simulink model "Echantillon"  (R2023b)
settings: Solver=VariableStepAuto  StartTime=0.0  StopTime=10.0  RelTol=1e-3
values from neighbouring files (symbols this model uses):
  C2 = retard/sysbod2(1 - retard)    [script_TD_asser_echantZdan.m]
  sysbod1 = c2d(sysbo , Te , 'foh')    [script_TD_asser_echantZdan.m]
libraries: slctrl_linear x1
settings Model: Creator=boris  LastModifiedBy=boris

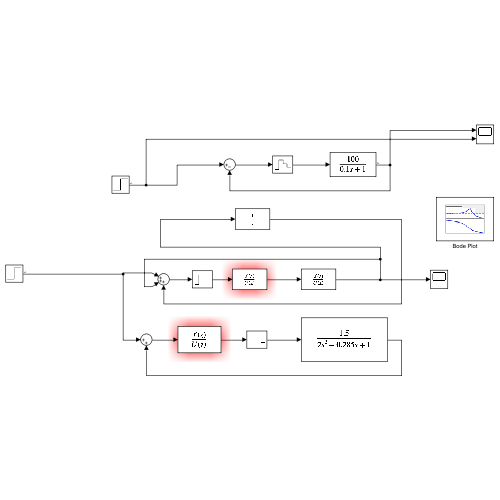
[thumbnail: Simulink's stored preview of the top-level diagram]
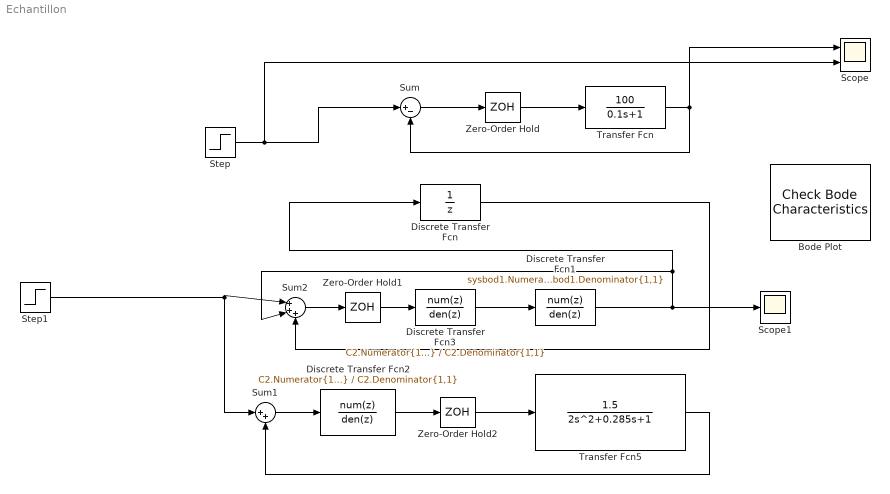
== system Echantillon ==
  Bode Plot : slctrl_linear/Check Bode  Characteristics  InstantiateOnLoad=on  SaveOperatingPoints=off  LinearizationIOs={}  LinearizeAt=SnapshotTimes  SnapshotTimes=[0]  TriggerType=rising  SampleTime=auto  RateConversionMethod=zoh  PreWarpFreq=10  UseExactDelayModel=off  UseFullBlockNameLabels=off  UseBusSignalLabels=off  enabled=on  stopWhenAssertionFail=off  export=off  ViewDlgPos=[]  OpenViewOnLoad=off  LaunchViewOnOpen=off  FrequencyUnits=rad/s  MagnitudeUnits=dB  PhaseUnits=deg  TimeUnits=seconds  EnableUpperBound=on  UpperBoundFrequencies=[]  UpperBoundMagnitudes=[]  EnableLowerBound=off  LowerBoundFrequencies=[]  LowerBoundMagnitudes=[]
      settings: LibrarySourceBlock=slctrlblks/Linear Analysis Plots/Bode Plot  SaveToWorkspace=off  SaveName=sys
  Discrete Transfer Fcn : DiscreteTransferFcn  Denominator=[1 0]
  Discrete Transfer Fcn1 : DiscreteTransferFcn  Numerator=sysbod1.Numerator{1,1}  Denominator=sysbod1.Denominator{1,1}
  Discrete Transfer Fcn2 : DiscreteTransferFcn  Numerator=C2.Numerator{1,1}  Denominator=C2.Denominator{1,1}
  Discrete Transfer Fcn3 : DiscreteTransferFcn  Numerator=C2.Numerator{1,1}  Denominator=C2.Denominator{1,1}
  Scope : Scope  NumInputPorts=2
  Scope1 : Scope
  Step : Step  After=10  SampleTime=0
  Step1 : Step  After=10  SampleTime=0
  Sum : Sum  Inputs=|+-
  Sum1 : Sum  Inputs=|++
  Sum2 : Sum  Inputs=|+++
  Transfer Fcn : TransferFcn  Numerator=[100]  Denominator=[0.1 1]
  Transfer Fcn5 : TransferFcn  Numerator=[1.5]  Denominator=[2 0.285 1]
  Zero-Order Hold : ZeroOrderHold  SampleTime=0.0001
  Zero-Order Hold1 : ZeroOrderHold  SampleTime=0.0001
  Zero-Order Hold2 : ZeroOrderHold  SampleTime=0.0001
  wires:
  Zero-Order Hold/1 -> Transfer Fcn/1
  Sum/1 -> Zero-Order Hold/1
  Transfer Fcn/1 -> Sum/2, Scope/1
  Step/1 -> Scope/2, Sum/1
  Step1/1 -> Sum2/1, Sum1/1
  Sum2/1 -> Zero-Order Hold1/1
  Zero-Order Hold1/1 -> Discrete Transfer Fcn3/1
  Sum1/1 -> Discrete Transfer Fcn2/1
  Discrete Transfer Fcn1/1 -> Scope1/1, Discrete Transfer Fcn/1, Sum2/2
  Discrete Transfer Fcn/1 -> Sum2/3
  Zero-Order Hold2/1 -> Transfer Fcn5/1
  Transfer Fcn5/1 -> Sum1/2
  Discrete Transfer Fcn3/1 -> Discrete Transfer Fcn1/1
  Discrete Transfer Fcn2/1 -> Zero-Order Hold2/1
